simulink model "CruiseCtrl_StateFeedback_Int"  (Simulink 10.1)
settings: Solver=ode45  StartTime=0.0  StopTime=40  MaxStep=0.01  RelTol=1e-3  EnableMultiTasking=on
values from neighbouring files (symbols this model uses):
  A = [[-1/tau 0];[1/m -rho*CD*Af*x2e/m]]    [CruiseCtrl_StateFeedback_Int_design.m]
  B1 = [B H]    [CruiseCtrl_StateFeedback_Int_design.m]
  C1 = eye(2)    [CruiseCtrl_StateFeedback_Int_design.m]
  D1 = zeros(2)    [CruiseCtrl_StateFeedback_Int_design.m]
  g = 9.82    [CruiseCtrl_StateFeedback_Int_design.m]
  Kaug = [0.0000 1.4349 0.4582]    [CruiseCtrl_StateFeedback_Int_design.m]
  ue = rw*x1e/k/r    (= 0.385125)    [CruiseCtrl_StateFeedback_Int_design.m]
  x1e = 0.5*rho*CD*Af*x2e^2+m*g*f    (= 6162)    [CruiseCtrl_StateFeedback_Int_design.m]
  x2e = 15    [CruiseCtrl_StateFeedback_Int_design.m]
settings Model: Creator=JonasMac  LastModifiedBy=Tomas
settings DataIOCC: LimitDataPoints=on
settings DebuggingCC: SolverPrmCheckMsg=warning
settings GRTTargetCC: CombineOutputUpdateFcns=on  GRTInterface=off

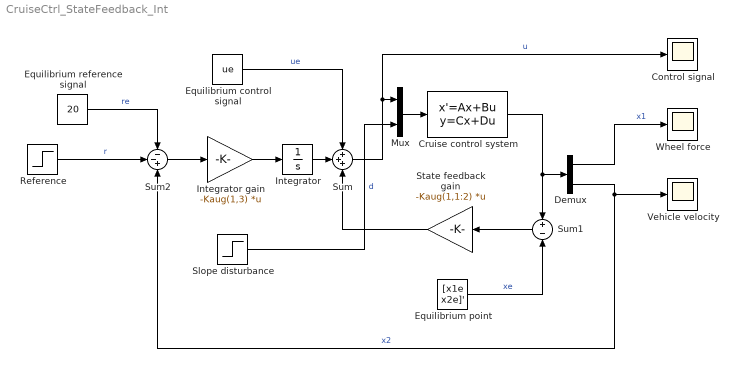
== system CruiseCtrl_StateFeedback_Int ==
  Control signal : Scope
  Cruise control system : StateSpace  A=A  B=B1  C=C1  D=D1
  Demux : Demux  Outputs=2
  Equilibrium control signal : Constant  Value=ue
  "Equilibrium point " : Constant  Value=[x1e x2e]'
  Equilibrium reference signal : Constant  Value=20
  Integrator : Integrator
  Integrator gain : Gain  Gain=-Kaug(1,3)  Multiplication=Matrix(K*u)
  Mux : Mux  Inputs=2
  Reference : Step  After=5  SampleTime=0
  Slope disturbance : Step  Time=20  After=g*sin(2*pi/180)  SampleTime=0
  State feedback gain : Gain  Gain=-Kaug(1,1:2)  Multiplication=Matrix(K*u)
  Sum : Sum  Inputs=+++
  Sum1 : Sum  Inputs=+-
  Sum2 : Sum  Inputs=--+
  Vehicle velocity : Scope
  Wheel force : Scope
  wires:
  Demux/1 -> Wheel force/1  "x1"
  Demux/2 -> Sum2/3, Vehicle velocity/1  "x2"
  Sum/1 -> Control signal/1, Mux/1  "u"
  Slope disturbance/1 -> Mux/2  "d"
  Integrator/1 -> Sum/2
  Equilibrium control signal/1 -> Sum/1  "ue"
  Cruise control system/1 -> Sum1/1, Demux/1
  Mux/1 -> Cruise control system/1
  State feedback gain/1 -> Sum/3
  Sum1/1 -> State feedback gain/1
  "Equilibrium point "/1 -> Sum1/2  "xe"
  Sum2/1 -> Integrator gain/1
  Integrator gain/1 -> Integrator/1
  Reference/1 -> Sum2/2  "r"
  Equilibrium reference signal/1 -> Sum2/1  "re"
